simulink model "task1"  (R2012b)
settings: Solver=ode45  StartTime=0.0  StopTime=10.0  RelTol=1e-3
settings Model: Creator=student-at  LastModifiedBy=student-at

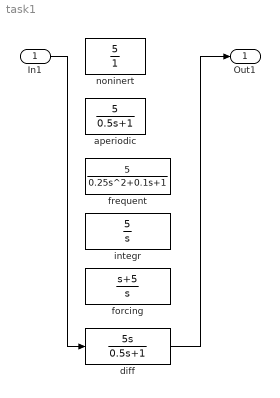
== system task1 ==
  In1 : Inport
  aperiodic : TransferFcn  Numerator=[5]  Denominator=[0.5 1]
  diff : TransferFcn  Numerator=[5 0]  Denominator=[0.5 1]
  forcing : TransferFcn  Numerator=[1 5]  Denominator=[1 0]
  frequent : TransferFcn  Numerator=[5]  Denominator=[0.25 0.1 1]
  integr : TransferFcn  Numerator=[5]  Denominator=[1 0]
  noninert : TransferFcn  Numerator=[5]  Denominator=[0 1]
  Out1 : Outport
  wires:
  In1/1 -> diff/1
  diff/1 -> Out1/1
